simulink subsystem "rp_dac"  (R2021a)
settings: Solver=VariableStepAuto  StartTime=0.0  StopTime=10.0  RelTol=1e-3
libraries: xbsIndex_r4 x4, xps_library x3
settings Model: Creator=casper  LastModifiedBy=casper

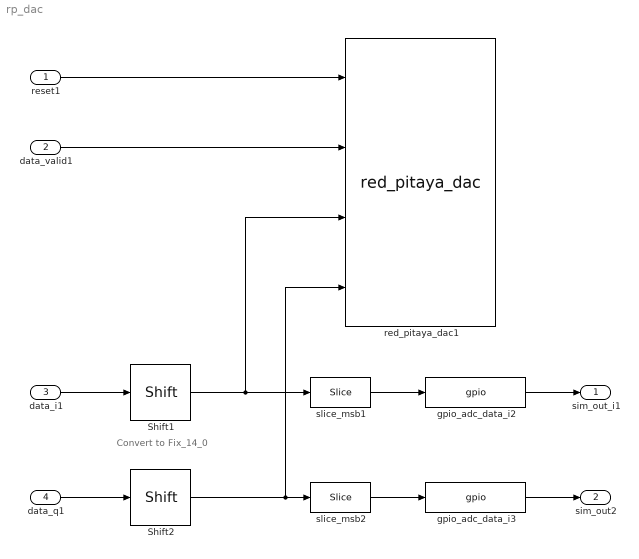
== system rp_dac ==
  note: Convert to Fix_14_0
  reset1 : Inport
  data_valid1 : Inport  Port=2
  data_i1 : Inport  Port=3
  data_q1 : Inport  Port=4
  Shift1 : xbsIndex_r4/Shift  shift_dir=Left  shift_bits=12  en=off  latency=1  precision=User Defined  arith_type="Signed  (2's comp)"  n_bits=14  bin_pt=0  quantization=Truncate  overflow=Wrap  dbl_ovrd=off  block_type=shift
  Shift2 : xbsIndex_r4/Shift  shift_dir=Left  shift_bits=12  en=off  latency=1  precision=User Defined  arith_type="Signed  (2's comp)"  n_bits=14  bin_pt=0  quantization=Truncate  overflow=Wrap  dbl_ovrd=off  block_type=shift
  gpio_adc_data_i2 : xps_library/IO/gpio  Tag=xps:gpio  io_group_params_forwarded=on  io_group=ROACH2:led  io_group_real=gpio  io_group_custom=0  io_dir=out  arith_type="Signed  (2's comp)"  bitwidth=8  bin_pt=0  bit_index=[0,1,2,3,4,5,6,7]  sample_period=1  use_single_ended=off  use_ddr=off  reg_iob=on  reg_clk_phase=0  termination=None  use_iodelay=off
      settings: SourceProductName=CASPER XPS Blockset
  gpio_adc_data_i3 : xps_library/IO/gpio  Tag=xps:gpio  io_group_params_forwarded=on  io_group=ROACH2:led  io_group_real=gpio  io_group_custom=0  io_dir=out  arith_type="Signed  (2's comp)"  bitwidth=8  bin_pt=0  bit_index=[8,9,10,11,12,13,14,15]  sample_period=1  use_single_ended=off  use_ddr=off  reg_iob=on  reg_clk_phase=0  termination=None  use_iodelay=off
      settings: SourceProductName=CASPER XPS Blockset
  red_pitaya_dac1 : xps_library/DACs/red_pitaya_dac  Tag=xps:red_pitaya_dac  bits=14
      settings: SourceProductName=CASPER XPS Blockset
  slice_msb1 : xbsIndex_r4/Slice  nbits=8  boolean_output=off  mode=Upper Bit Location + Width  bit1=0  base1=MSB of Input  bit0=0  base0=LSB of Input  dbl_ovrd=off  block_type=slice
  slice_msb2 : xbsIndex_r4/Slice  nbits=8  boolean_output=off  mode=Upper Bit Location + Width  bit1=0  base1=MSB of Input  bit0=0  base0=LSB of Input  dbl_ovrd=off  block_type=slice
  sim_out_i1 : Outport
  sim_out2 : Outport  Port=2
  wires:
  gpio_adc_data_i3/1 -> sim_out2/1
  data_q1/1 -> Shift2/1
  slice_msb2/1 -> gpio_adc_data_i3/1
  data_valid1/1 -> red_pitaya_dac1/2
  gpio_adc_data_i2/1 -> sim_out_i1/1
  Shift2/1 -> red_pitaya_dac1/4, slice_msb2/1
  slice_msb1/1 -> gpio_adc_data_i2/1
  data_i1/1 -> Shift1/1
  reset1/1 -> red_pitaya_dac1/1
  Shift1/1 -> red_pitaya_dac1/3, slice_msb1/1
